simulink model "ACCMod001"  (Simulink 8.3)
settings: Solver=ode45  StartTime=0.0  StopTime=10.0  RelTol=1e-3
model workspace (MAT data in the model file):
  pACC.Kp = 0.5
  pACC.minDist2Target = 50
  pACC.avgACCactiveTime = 20
  pACC.LearnGain = 5
  pACC.Ki = 1e-05
  pACC.KpDist = 1
  pACC.KiDist = 0.01
  pACC.SampleTime = 0.1
  pACC.ACCBuffer : numeric (value not decoded)
settings Model: Creator=swami  LastModifiedBy=swami
settings SolverCC: AutoInsertRateTranBlk=on
settings DataIOCC: SignalLoggingSaveFormat=Dataset
settings DebuggingCC: UnderspecifiedInitializationDetection=Simplified  StateNameClashWarn=none
settings GRTTargetCC: CombineOutputUpdateFcns=on  GRTInterface=off

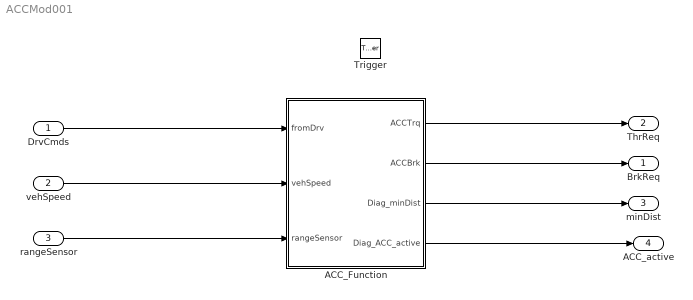
== system ACCMod001 ==
  DrvCmds : Inport  PortDimensions=4
  vehSpeed : Inport  Port=2
  rangeSensor : Inport  Port=3
  Trigger : TriggerPort  TriggerType=function-call  PortDimensions=1
  ACC_Function : MATLAB Function  TreatAsAtomicUnit=on
  BrkReq : Outport  PortDimensions=1  InitialOutput=0
  ThrReq : Outport  Port=2  PortDimensions=1  InitialOutput=0
  minDist : Outport  Port=3  PortDimensions=1  InitialOutput=50
  ACC_active : Outport  Port=4  PortDimensions=1  InitialOutput=0
  wires:
  ACC_Function/1(ACCTrq) -> ThrReq/1
  ACC_Function/2(ACCBrk) -> BrkReq/1
  ACC_Function/3(Diag_minDist) -> minDist/1
  ACC_Function/4(Diag_ACC_active) -> ACC_active/1
  DrvCmds/1 -> ACC_Function/1(fromDrv)
  vehSpeed/1 -> ACC_Function/2(vehSpeed)
  rangeSensor/1 -> ACC_Function/3(rangeSensor)

== matlab function ACC_Function ==
  settings: sampleTime=0.1
  data: fromDrv input double; ACCTrq output double; ACCBrk output double; vehSpeed input double; rangeSensor input double; pACC parameter double; Diag_minDist output double; Diag_ACC_active output double
function [ACCTrq,ACCBrk,Diag_minDist, Diag_ACC_active] = fcn(fromDrv,vehSpeed,rangeSensor,pACC)
%#codegen
persistent CC_active;
persistent ACC_active;
persistent ACC_starttime;
persistent minDist2TargetLearn;
persistent intClk;
persistent torq_req_int;
persistent torq_req_old;
persistent errorKiDist;
if isempty(ACC_active)
    ACC_active = 0;
    minDist2TargetLearn = 0;
    ACC_starttime = 0; % would like to avaoid this
    intClk = 0;
    CC_active = 0;
    torq_req_int = 0;
    torq_req_old = 0;
    errorKiDist = 0;
end
SampleTime = 0.1;
intClk = intClk + SampleTime;
ACC_active_old = ACC_active;
CC_active_old = CC_active;

deltaSpeedDesd = 0;

clktime = intClk;

DrvBrk = fromDrv(1);
DrvThr = fromDrv(2);
DrvCCSw = fromDrv(3);
DrvCCSetPoint = fromDrv(4);

dist2Target = rangeSensor(1);

minDist2Target = pACC.minDist2Target + minDist2TargetLearn;
KpDist = pACC.KpDist;
ACCBuffer = minDist2Target * 0.9;


if DrvCCSw > 0.5
    if (CC_active == 0)
        CC_active = 1;
    end
    if (dist2Target < minDist2Target)
        % need to slow down
        ACC_active = 1;
    else
        ACC_active = 0;
    end
    
    if (ACC_active == 1)
        errorKpDist = (dist2Target - minDist2Target) * pACC.KpDist;
        errorKiDist = errorKiDist + errorKpDist * pACC.KiDist;
        deltaSpeedDesd = errorKpDist + errorKiDist;
        if (deltaSpeedDesd > 0.0)
            deltaSpeedDesd = 0;
            ACC_active = 0;
        end
    else
        deltaSpeedDesd = 0;
    end
    
    errorKp = (DrvCCSetPoint + deltaSpeedDesd - vehSpeed)* pACC.Kp;

    
   torq_req_int = torq_req_int + errorKp * pACC.Ki;    
   torq_req_prop = errorKp;   
   torq_req = torq_req_prop + torq_req_int;
       
   if (torq_req > 1.0)
       torq_req = 1.0;
   elseif (torq_req < -1.0)
       torq_req = -1.0;
   end    
   if torq_req < 0.0
       ACCBrk = 0.0 - torq_req;
       ACCTrq = 0.0;
   else
       ACCBrk = 0.0;
       ACCTrq = torq_req;
   end
else
    CC_active = 0;
    ACCTrq = DrvThr;
    ACCBrk = DrvBrk;
    torq_req = ACCTrq;
end

if ((CC_active_old ==0) && (CC_active == 1))
    torq_req_int = torq_req_old
end



if ((ACC_active_old == 0) && (ACC_active == 1))
    ACC_starttime = clktime;
    errorKiDist = 0;
    torq_req_int = torq_req_old;
end

torq_req_old = torq_req;


%check if this is start of ACC turn off
if ((ACC_active_old == 1) && (ACC_active == 0))
    if (clktime - ACC_starttime) < pACC.avgACCactiveTime
        minDist2TargetLearn = minDist2TargetLearn + pACC.LearnGain;
    end
end

Diag_minDist = minDist2Target;
Diag_ACC_active = ACC_active;
